simulink model "PI_controller"  (R2024a)
settings: Solver=VariableStepAuto  StartTime=0.0  StopTime=10.0  RelTol=1e-3
undefined symbols (not defined in the file): detect_delay, Gd, gear, Gn, Kp, tau, Wrad
settings Model: Creator=Emil  LastModifiedBy=lukas

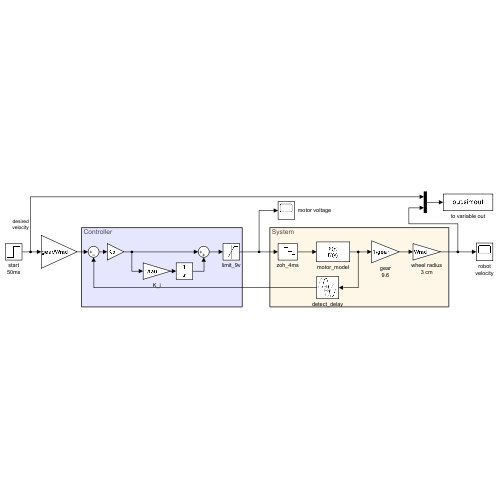
[thumbnail: Simulink's stored preview of the top-level diagram]
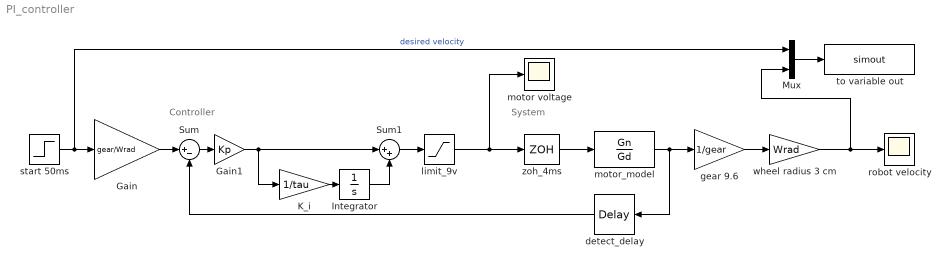
== system PI_controller ==
  note: System
  note: Controller
  Gain : Gain  Gain=gear/Wrad
  Gain1 : Gain  Gain=Kp
  Integrator : Integrator
  K_i : Gain  Gain=1/tau
  Mux : Mux  Inputs=2
  Sum : Sum  Inputs=|+-
  Sum1 : Sum  Inputs=|++
  detect_delay : TransportDelay  DelayTime=detect_delay
  gear 9.6 : Gain  Gain=1/gear
  limit_9v : Saturate  UpperLimit=9  LowerLimit=-9
  motor voltage : Scope
  motor_model : TransferFcn  Numerator=Gn  Denominator=Gd
  robot velocity : Scope
  start 50ms : Step  Time=0.05  After=1.2  SampleTime=0
  to variable out : ToWorkspace  VariableName=simout  SaveFormat=Timeseries  SampleTime=-1
  wheel radius 3 cm : Gain  Gain=Wrad
  zoh_4ms : ZeroOrderHold  SampleTime=-1
  wires:
  start 50ms/1 -> Gain/1, Mux/1  "desired velocity"
  Gain/1 -> Sum/1
  Sum/1 -> Gain1/1
  limit_9v/1 -> zoh_4ms/1, motor voltage/1
  zoh_4ms/1 -> motor_model/1
  motor_model/1 -> gear 9.6/1, detect_delay/1
  detect_delay/1 -> Sum/2
  gear 9.6/1 -> wheel radius 3 cm/1
  wheel radius 3 cm/1 -> Mux/2, robot velocity/1
  Mux/1 -> to variable out/1
  Sum1/1 -> limit_9v/1
  Gain1/1 -> K_i/1, Sum1/1
  K_i/1 -> Integrator/1
  Integrator/1 -> Sum1/2
